simulink model "Multidifusor2"  (R2023a)
settings: Solver=VariableStepAuto  StartTime=0.0  StopTime=10.0  RelTol=1e-3
settings Model: Creator=santi  LastModifiedBy=santi

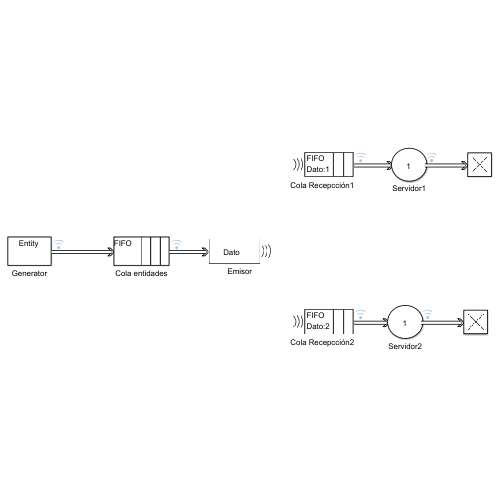
[thumbnail: Simulink's stored preview of the top-level diagram]
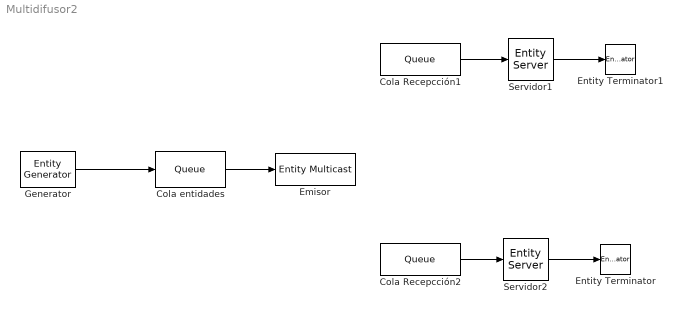
== system Multidifusor2 ==
  Cola Recepcción1 : Queue  OutputPortMessageModes=m  Capacity=5  EntityArrivalSource=Multicast  MulticastTag=Dato
  Cola Recepcción2 : Queue  OutputPortMessageModes=m  Capacity=5  EntityArrivalSource=Multicast  MulticastTag=Dato
  Cola entidades : Queue  InputPortMessageModes=m  OutputPortMessageModes=m
  Emisor : EntityMulticast  Tag=Dato  InputPortMessageModes=m  MulticastTag=Dato
  Entity Terminator : EntityTerminator  InputPortMessageModes=m
  Entity Terminator1 : EntityTerminator  InputPortMessageModes=m
  Generator : EntityGenerator  OutputPortMessageModes=m  TimeSource=MATLAB action  EntityType=Structured  EntityTypeName=Entity
  Servidor1 : EntityServer  InputPortMessageModes=m  OutputPortMessageModes=m  Capacity=1
  Servidor2 : EntityServer  InputPortMessageModes=m  OutputPortMessageModes=m  Capacity=1
  wires:
  Generator/1 -> Cola entidades/1
  Cola entidades/1 -> Emisor/1
  Cola Recepcción2/1 -> Servidor2/1
  Servidor2/1 -> Entity Terminator/1
  Servidor1/1 -> Entity Terminator1/1
  Cola Recepcción1/1 -> Servidor1/1
